simulink model "Sanboks_SIMULINK_v0_4"  (R2021a)
settings: Solver=ode45  StartTime=0  StopTime=1600  FixedStep=1  RelTol=1e-4
InitFcn:
  | Acc_x=0;
undefined symbols (not defined in the file): achievable_velocity, air_density, car_mass, center_of_gravity, coefficient_rolling_resistance, conti_PID, conti_rpm, conti_torque, current, distance, drag_coefficient, final_drivetrain_efficiency, front_braking_torque, front_frequency, front_motion_ratio, front_tire_rate, front_trackwidth, frontal_area, gear_ratio, grade_of_track, gravity, h1f, h1r, hf, hr, long_friction, no_laps, no_of_motors, peak_PID, peak_rpm, peak_torque, Rear_braking_torque, rear_frequency, rear_motion_ratio, rear_tire_rate, rear_trackwidth, rear_weight_distribution, reference_steering_angle, rho, rot_mass, start_time_for_peak, steering_ratio, supply_voltage, tire_radius, track_length, wheelbase, x_leng
libraries: simulink x2, pid_lib x2
settings Model: Creator=Swapnil Mane  LastModifiedBy=rk
settings SolverCC: MaxConsecutiveMinStep=auto  ZeroCrossAlgorithm=Adaptive  AlgebraicLoopSolver=TrustRegion  SolverResetMethod=Robust
settings DebuggingCC: AlgebraicLoopMsg=none  MaskedZcDiagnostic=none  IgnoredZcDiagnostic=none  SFMachineParentedDataDiag=warning

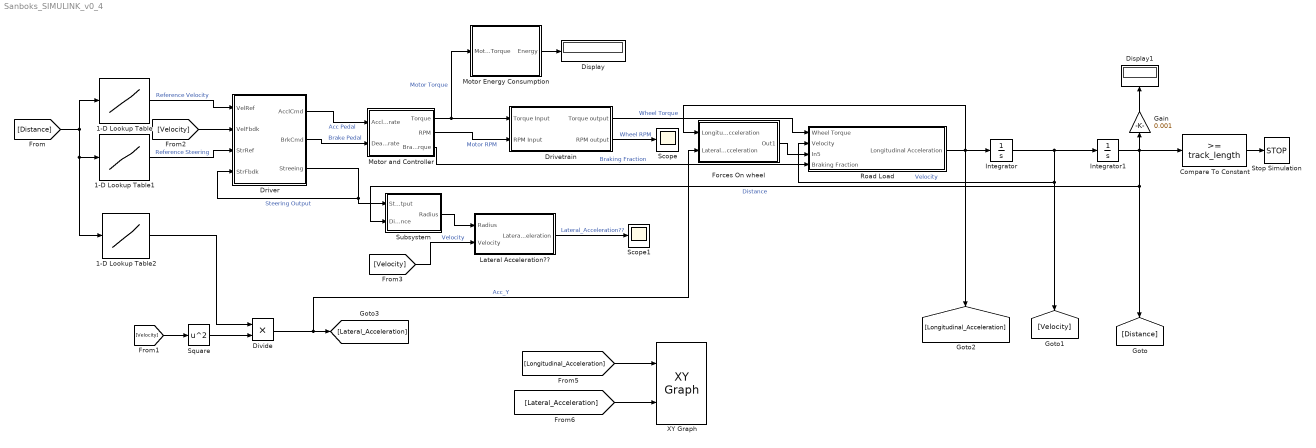
== system Sanboks_SIMULINK_v0_4 ==
  1-D Lookup Table : Lookup_n-D  NumberOfTableDimensions=1  BreakpointsForDimension1=distance(1:2:x_leng*no_laps)  Table=achievable_velocity  InternalRulePriority=Speed  RndMeth=Simplest  InputSameDT=on
  1-D Lookup Table1 : Lookup_n-D  NumberOfTableDimensions=1  BreakpointsForDimension1=distance(1:x_leng*no_laps)  Table=reference_steering_angle  InternalRulePriority=Speed  RndMeth=Simplest  InputSameDT=on
  1-D Lookup Table2 : Lookup_n-D  NumberOfTableDimensions=1  BreakpointsForDimension1=distance(1:2:x_leng*no_laps)  Table=rho  InternalRulePriority=Speed  RndMeth=Simplest  InputSameDT=on
  Compare To Constant : simulink/Logic and Bit Operations/Compare To Constant  relop=>=  const=track_length  OutDataTypeStr=boolean
  Display : Display
  Display1 : Display
  Divide : Product  Inputs=**
  Driver : Subsystem
      mask Display: image('$imagefile'); % Use "Edit Image" on toolstrip to change.
  Drivetrain : Subsystem
      mask Display: image('$imagefile'); % Use "Edit Image" on toolstrip to change.
  Forces On wheel : Subsystem
  Gain : Gain  Gain=0.001
  Integrator : Integrator
  Integrator1 : Integrator
  Lateral Acceleration?? : Subsystem
  Motor Energy Consumption : Subsystem
  Motor and Controller : Subsystem
      mask Display: image('$imagefile'); % Use "Edit Image" on toolstrip to change.
  Road Load : Subsystem
  Scope : Scope
  Scope1 : Scope
  Square : Math  Operator=square  SaturateOnIntegerOverflow=on
  Stop Simulation : Stop
  Subsystem : Subsystem
  XY Graph : simulink/Sinks/XY Graph  xmin=-20  xmax=20  ymin=-20  ymax=20  st=-1
  wires:
  Driver/1(AcclCmd) -> Motor and Controller/1(Acclerate)  "Acc Pedal"
  Motor and Controller/1(Torque) -> Drivetrain/1(Torque Input), Motor Energy Consumption/1(Motor Torque)  "Motor Torque"
  Motor and Controller/2(" RPM") -> Drivetrain/2(RPM Input)  "Motor RPM"
  Driver/2(BrkCmd) -> Motor and Controller/2(Deaccelerate)  "Brake Pedal"
  Compare To Constant/1 -> Stop Simulation/1
  Integrator1/1 -> Compare To Constant/1, Gain/1, [Distance], Subsystem/2(Distance)  "Distance"
  1-D Lookup Table/1 -> Driver/1(VelRef)  "Reference Velocity"
  Integrator/1 -> Integrator1/1, Road Load/2(Velocity), [Velocity]  "Velocity"
  1-D Lookup Table1/1 -> Driver/3(StrRef)  "Reference Steering"
  Driver/3(Streeing) -> Driver/4(StrFbdk), Subsystem/1(Steering Output)  "Steering Output"
  [Velocity] -> Driver/2(VelFbdk)
  [Velocity] -> Lateral Acceleration??/2(Velocity)  "Velocity"
  [Lateral_Acceleration] -> XY Graph/2
  [Longitudinal_Acceleration] -> XY Graph/1
  Subsystem/1(Radius) -> Lateral Acceleration??/1(Radius)
  Motor Energy Consumption/1(Energy) -> Display/1
  Drivetrain/2(RPM output) -> Scope/1  "Wheel RPM"
  [Distance] -> 1-D Lookup Table2/1, 1-D Lookup Table1/1, 1-D Lookup Table/1
  Gain/1 -> Display1/1
  Road Load/1(Longitudinal Acceleration) -> Forces On wheel/1(Longitunal Acceleration), [Longitudinal_Acceleration], Integrator/1
  Drivetrain/1(Torque output) -> Road Load/1(Wheel Torque)  "Wheel Torque"
  Forces On wheel/1(Out1) -> Road Load/3(In5)
  Motor and Controller/3(Braking Torque) -> Road Load/4(Braking Fraction)  "Braking Fraction"
  1-D Lookup Table2/1 -> Divide/1
  [Velocity] -> Square/1
  Square/1 -> Divide/2
  Divide/1 -> Forces On wheel/2(Lateral_Acceleration), [Lateral_Acceleration]  "Acc_Y"
  Lateral Acceleration??/1(Lateral_Acceleration) -> Scope1/1  "Lateral_Acceleration??"

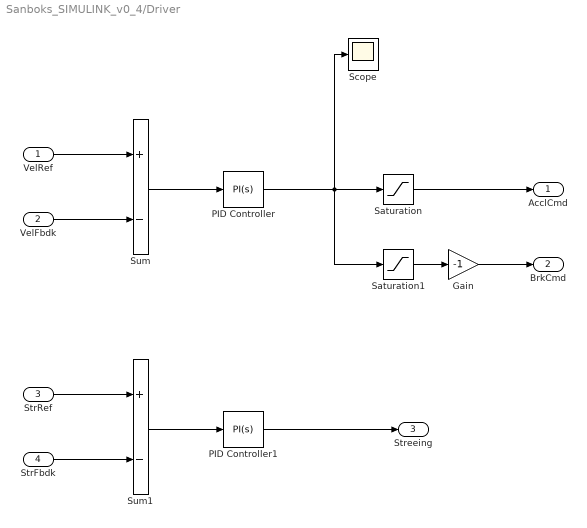
== system Sanboks_SIMULINK_v0_4/Driver ==
  VelRef : Inport
  VelFbdk : Inport  Port=2
  StrRef : Inport  Port=3
  StrFbdk : Inport  Port=4
  Gain : Gain  Gain=-1
  PID Controller : pid_lib/PID Controller  Controller=PI  Form=Parallel  TimeDomain=Continuous-time  UseExternalTs=off  SampleTime=-1  IntegratorMethod=Forward Euler  FilterMethod=Forward Euler  ControllerParametersSource=internal  P=1  I=0  D=0  UseFilter=on  N=10  TunerSelectOption=Transfer Function Based (PID Tuner App)  InitialConditionSource=internal  InitialConditionForIntegrator=0  InitialConditionForFilter=0  DifferentiatorICPrevScaledInput=0  ExternalReset=none  TrackingMode=off  Kt=1  LimitOutput=off  SatLimitsSource=internal  UpperSaturationLimit=inf  LowerSaturationLimit=-inf  LinearizeAsGain=on  AntiWindupMode=none  Kb=1  POutMin=[]  POutMax=[]  IOutMin=[]  IOutMax=[]  DOutMin=[]  DOutMax=[]  NOutMin=[]  NOutMax=[]  SumOutMin=[]  SumOutMax=[]  SaturationOutMin=[]  SaturationOutMax=[]  PParamMin=[]  PParamMax=[]  IParamMin=[]  IParamMax=[]  DParamMin=[]  DParamMax=[]  NParamMin=[]  NParamMax=[]  KbParamMin=[]  KbParamMax=[]  KtParamMin=[]  KtParamMax=[]  KbOutMin=[]  KbOutMax=[]  KtOutMin=[]  KtOutMax=[]  IntegratorOutMin=[]  IntegratorOutMax=[]  FilterOutMin=[]  FilterOutMax=[]  SumI1OutMin=[]  SumI1OutMax=[]  SumI2OutMin=[]  SumI2OutMax=[]  SumI3OutMin=[]  SumI3OutMax=[]  SumI4OutMin=[]  SumI4OutMax=[]  SumDOutMin=[]  SumDOutMax=[]  DifferentiatorOutMin=[]  DifferentiatorOutMax=[]  FilterDiffOutCoefMin=[]  FilterDiffOutCoefMax=[]  ReciprocalOutMin=[]  ReciprocalOutMax=[]  SumDenOutMin=[]  SumDenOutMax=[]  SumNumOutMin=[]  SumNumOutMax=[]  DivideOutMin=[]  DivideOutMax=[]  UdiffTsProdOutMin=[]  UdiffTsProdOutMax=[]  NTsProdOutMin=[]  NTsProdOutMax=[]  UintegralTsProdOutMin=[]  UintegralTsProdOutMax=[]  UngainTsProdOutMin=[]  UngainTsProdOutMax=[]  IntegratorContinuousStateAttributes=''  IntegratorStateMustResolveToSignalObject=off  IntegratorRTWStateStorageClass=Auto  FilterContinuousStateAttributes=''  FilterStateMustResolveToSignalObject=off  FilterRTWStateStorageClass=Auto  ParallelPVariant=InternalParameters  IdealPVariant=Disabled  IVariant=InternalParameters  DVariant=Disabled  IntegratorVariant=Continuous  SatVariant=Disabled  AWVariant=Passthrough  PCopyVariant=Disabled  TRVariant=Disabled  FdbkBlocksVariant=Forward  IdealPFdbkVariant=Disabled  SatFdbkVariant=Disabled  DerivativeFilterVariant=Disabled  NVariant=Disabled  NCopyVariant=Disabled_SignalSpec  FilterICVariant=Disabled  IntegratorICVariant=InternalICs  ExternalResetVariant=Disabled  TRSumVariant=Passthrough  SumFdbkVariant=Disabled  SumVariant=Sum_PI  TsampFilterVariant=InternalTs  TsampNgainVariant=Passthrough  TsampIntegralVariant=Passthrough  ExternalSaturationOutDataTypeStr=Inherit: Same as second input
  PID Controller1 : pid_lib/PID Controller  Controller=PI  Form=Parallel  TimeDomain=Continuous-time  UseExternalTs=off  SampleTime=-1  IntegratorMethod=Forward Euler  FilterMethod=Forward Euler  ControllerParametersSource=internal  P=2  I=1  D=0  UseFilter=on  N=10  TunerSelectOption=Transfer Function Based (PID Tuner App)  InitialConditionSource=internal  InitialConditionForIntegrator=0  InitialConditionForFilter=0  DifferentiatorICPrevScaledInput=0  ExternalReset=none  TrackingMode=off  Kt=1  LimitOutput=off  SatLimitsSource=internal  UpperSaturationLimit=inf  LowerSaturationLimit=-inf  LinearizeAsGain=on  AntiWindupMode=none  Kb=1  POutMin=[]  POutMax=[]  IOutMin=[]  IOutMax=[]  DOutMin=[]  DOutMax=[]  NOutMin=[]  NOutMax=[]  SumOutMin=[]  SumOutMax=[]  SaturationOutMin=[]  SaturationOutMax=[]  PParamMin=[]  PParamMax=[]  IParamMin=[]  IParamMax=[]  DParamMin=[]  DParamMax=[]  NParamMin=[]  NParamMax=[]  KbParamMin=[]  KbParamMax=[]  KtParamMin=[]  KtParamMax=[]  KbOutMin=[]  KbOutMax=[]  KtOutMin=[]  KtOutMax=[]  IntegratorOutMin=[]  IntegratorOutMax=[]  FilterOutMin=[]  FilterOutMax=[]  SumI1OutMin=[]  SumI1OutMax=[]  SumI2OutMin=[]  SumI2OutMax=[]  SumI3OutMin=[]  SumI3OutMax=[]  SumI4OutMin=[]  SumI4OutMax=[]  SumDOutMin=[]  SumDOutMax=[]  DifferentiatorOutMin=[]  DifferentiatorOutMax=[]  FilterDiffOutCoefMin=[]  FilterDiffOutCoefMax=[]  ReciprocalOutMin=[]  ReciprocalOutMax=[]  SumDenOutMin=[]  SumDenOutMax=[]  SumNumOutMin=[]  SumNumOutMax=[]  DivideOutMin=[]  DivideOutMax=[]  UdiffTsProdOutMin=[]  UdiffTsProdOutMax=[]  NTsProdOutMin=[]  NTsProdOutMax=[]  UintegralTsProdOutMin=[]  UintegralTsProdOutMax=[]  UngainTsProdOutMin=[]  UngainTsProdOutMax=[]  IntegratorContinuousStateAttributes=''  IntegratorStateMustResolveToSignalObject=off  IntegratorRTWStateStorageClass=Auto  FilterContinuousStateAttributes=''  FilterStateMustResolveToSignalObject=off  FilterRTWStateStorageClass=Auto  ParallelPVariant=InternalParameters  IdealPVariant=Disabled  IVariant=InternalParameters  DVariant=Disabled  IntegratorVariant=Continuous  SatVariant=Disabled  AWVariant=Passthrough  PCopyVariant=Disabled  TRVariant=Disabled  FdbkBlocksVariant=Forward  IdealPFdbkVariant=Disabled  SatFdbkVariant=Disabled  DerivativeFilterVariant=Disabled  NVariant=Disabled  NCopyVariant=Disabled_SignalSpec  FilterICVariant=Disabled  IntegratorICVariant=InternalICs  ExternalResetVariant=Disabled  TRSumVariant=Passthrough  SumFdbkVariant=Disabled  SumVariant=Sum_PI  TsampFilterVariant=InternalTs  TsampNgainVariant=Passthrough  TsampIntegralVariant=Passthrough  ExternalSaturationOutDataTypeStr=Inherit: Same as second input
  Saturation : Saturate  UpperLimit=1  LowerLimit=0
  Saturation1 : Saturate  UpperLimit=0  LowerLimit=-1
  Scope : Scope
  Sum : Sum  Inputs=+-
  Sum1 : Sum  Inputs=+-
  AcclCmd : Outport
  BrkCmd : Outport  Port=2
  Streeing : Outport  Port=3
  wires:
  PID Controller/1 -> Saturation1/1, Saturation/1, Scope/1
  VelFbdk/1 -> Sum/2
  Sum/1 -> PID Controller/1
  VelRef/1 -> Sum/1
  Saturation/1 -> AcclCmd/1
  Gain/1 -> BrkCmd/1
  Saturation1/1 -> Gain/1
  StrRef/1 -> Sum1/1
  Sum1/1 -> PID Controller1/1
  StrFbdk/1 -> Sum1/2
  PID Controller1/1 -> Streeing/1

== system Sanboks_SIMULINK_v0_4/Drivetrain ==
  Torque Input : Inport
  RPM Input : Inport  Port=2
  Divide : Product  Inputs=**/
  Divide1 : Product  Inputs=***
  Final Drivetrain Efficiency : Constant  Value=final_drivetrain_efficiency
  Gear Ratio : Constant  Value=gear_ratio
  Torque output : Outport
  RPM output : Outport  Port=2
  wires:
  Gear Ratio/1 -> Divide/3, Divide1/1
  Final Drivetrain Efficiency/1 -> Divide1/3, Divide/1
  RPM Input/1 -> Divide/2
  Divide/1 -> RPM output/1
  Torque Input/1 -> Divide1/2
  Divide1/1 -> Torque output/1

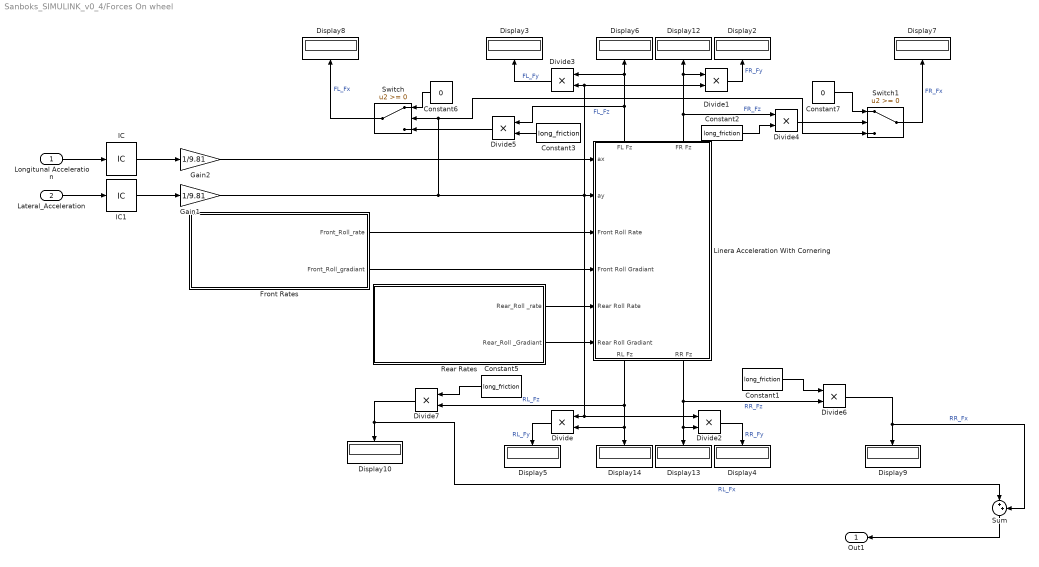
== system Sanboks_SIMULINK_v0_4/Forces On wheel ==
  Longitunal Acceleration : Inport
  Lateral_Acceleration : Inport  Port=2
  Constant{1..3,5} (4 alike) : Constant  Value=long_friction
  Constant6 : Constant  Value=0
  Constant7 : Constant  Value=0
  Display{2..10,12..14} (12 alike) : Display
  Divide{,1..7} (8 alike) : Product  Inputs=**
  Front Rates : Subsystem
  Gain1 : Gain  Gain=1/9.81
  Gain2 : Gain  Gain=1/9.81
  IC : InitialCondition  Value=0
  IC1 : InitialCondition  Value=0
  Linera Acceleration With Cornering : Subsystem
      settings: PortSchema="{\"entries\":[{\"content\":{\"sides\":[{\"content\":{\"connectorIds\":[\"In1\",\"In2\",\"In3\",\"In4\",\"In5\",\"In6\"]},\"type\":\"ConnectorPlacement.EquallySpacedRectSide\",\"uuid\":\"d773b041-193b-40c1-84f4-1820b4697a0f\"},{\"content\":{\"connectorIds\":[],\"side\":\"RIGHT\"},\"type\":\"ConnectorPlacement.EquallySpacedRectSide\",\"uuid\":\"63078260-0e7d-46b5-b894-dfb0cdd11ba9\"},{\"content\":{\"connectorIds\":[\"Out3\",\"Out4\"],\"side\":\"TOP\"},\"type\":\"ConnectorPlacement.EquallySpacedRectSide\",\"uuid\":\"e8ba9282-0130-45e1-8a34-44ae52181d51\"},{\"content\":{\"connectorIds\":[\"Out1\",\"Out2\"],\"side\":\"BOTTOM\"},\"type\":\"ConnectorPlacement.EquallySpacedRectSide\",\"uuid\":\"5bbf88fe-c1d3-4396-8228-1f5368518a99\"},{\"content\":{\"connectorIds\":[],\"side\":\"HIDDEN\"},\"type\":\"ConnectorPlacement.EquallySpacedRectSide\",\"uuid\":\"f592c54a-f6c6-4a08-a46d-6911c26235f2\"}]},\"type\":\"ConnectorPlacement.EquallySpacedConnector\",\"uuid\":\"5d9b9e8e-da8b-47d2-a239-b5c86b3b0142\"}],\"packageUris\":[\"http://schema.mathworks.com/mf0/Connector/R2020b\"],\"version\":\"1.0\"}"
  Rear Rates : Subsystem
  Sum : Sum  Inputs=|++
  Switch : Switch
  Switch1 : Switch
  Out1 : Outport
  wires:
  Switch1/1 -> Display7/1  "FR_Fx"
  Constant2/1 -> Divide4/2
  Constant3/1 -> Divide5/2
  Linera Acceleration With Cornering/2(RR Fz) -> Divide6/2, Divide2/2, Display13/1  "RR_Fz"
  Front Rates/1(Front_Roll_rate) -> Linera Acceleration With Cornering/3(Front Roll Rate)
  Divide6/1 -> Sum/2, Display9/1  "RR_Fx"
  Front Rates/2(Front_Roll_gradiant) -> Linera Acceleration With Cornering/4(Front Roll Gradiant)
  Gain1/1 -> Switch1/2, Switch/2, Linera Acceleration With Cornering/2(ay), Divide3/2, Divide1/2, Divide2/1, Divide/1
  Rear Rates/2(Rear_Roll _Gradiant) -> Linera Acceleration With Cornering/6(Rear Roll Gradiant)
  Divide1/1 -> Display2/1  "FR_Fy"
  Linera Acceleration With Cornering/1(RL Fz) -> Divide7/2, Divide/2, Display14/1  "RL_Fz"
  Divide5/1 -> Switch/3
  Constant5/1 -> Divide7/1
  Rear Rates/1(Rear_Roll _rate) -> Linera Acceleration With Cornering/5(Rear Roll Rate)
  Linera Acceleration With Cornering/3(" FL Fz") -> Divide5/1, Display6/1, Divide3/1  "FL_Fz"
  Divide4/1 -> Switch1/3
  Divide7/1 -> Display10/1, Sum/1  "RL_Fx"
  Linera Acceleration With Cornering/4(FR Fz) -> Divide1/1, Display12/1, Divide4/1  "FR_Fz"
  Gain2/1 -> Linera Acceleration With Cornering/1(ax)
  Divide3/1 -> Display3/1  "FL_Fy"
  Constant1/1 -> Divide6/1
  Divide/1 -> Display5/1  "RL_Fy"
  Constant6/1 -> Switch/1
  Divide2/1 -> Display4/1  "RR_Fy"
  Sum/1 -> Out1/1
  Switch/1 -> Display8/1  "FL_Fx"
  Constant7/1 -> Switch1/1
  IC/1 -> Gain2/1
  IC1/1 -> Gain1/1
  Longitunal Acceleration/1 -> IC/1
  Lateral_Acceleration/1 -> IC1/1

== system Sanboks_SIMULINK_v0_4/Lateral Acceleration?? ==
  Radius : Inport
  Velocity : Inport  Port=2
  Divide2 : Product  Inputs=**/
  Scope13 : Scope
  Lateral_Acceleration : Outport
  wires:
  Divide2/1 -> Lateral_Acceleration/1, Scope13/1
  Radius/1 -> Divide2/3
  Velocity/1 -> Divide2/2, Divide2/1

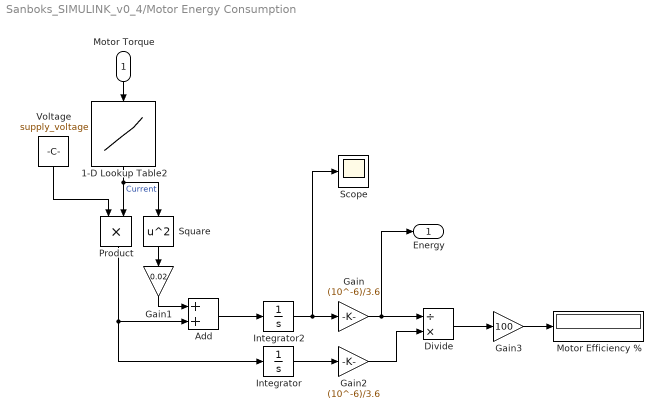
== system Sanboks_SIMULINK_v0_4/Motor Energy Consumption ==
  Motor Torque : Inport
  1-D Lookup Table2 : Lookup_n-D  NumberOfTableDimensions=1  BreakpointsForDimension1=peak_torque  Table=current  InternalRulePriority=Speed  RndMeth=Simplest  InputSameDT=on
  Add : Sum
  Divide : Product  Inputs=/*
  Gain : Gain  Gain=(10^-6)/3.6
  Gain1 : Gain  Gain=0.02
  Gain2 : Gain  Gain=(10^-6)/3.6
  Gain3 : Gain  Gain=100
  Integrator : Integrator
  Integrator2 : Integrator
  Motor Efficiency % : Display
  Product : Product
  Scope : Scope
  Square : Math  Operator=square  SaturateOnIntegerOverflow=on
  Voltage : Constant  Value=supply_voltage
  Energy : Outport
  wires:
  Product/1 -> Integrator/1, Add/2
  Gain1/1 -> Add/1
  Voltage/1 -> Product/1
  Add/1 -> Integrator2/1
  1-D Lookup Table2/1 -> Product/2, Square/1  "Current"
  Integrator2/1 -> Scope/1, Gain/1
  Motor Torque/1 -> 1-D Lookup Table2/1
  Gain/1 -> Energy/1, Divide/1
  Square/1 -> Gain1/1
  Integrator/1 -> Gain2/1
  Gain2/1 -> Divide/2
  Divide/1 -> Gain3/1
  Gain3/1 -> Motor Efficiency %/1

== system Sanboks_SIMULINK_v0_4/Motor and Controller ==
  Acclerate : Inport
  Deaccelerate : Inport  Port=2
  Motor : Subsystem
  Motor Controller : Subsystem
  Scope : Scope
  Torque : Outport
  " RPM" : Outport  Port=2
  Braking Torque : Outport  Port=3
  wires:
  Acclerate/1 -> Motor Controller/1(Acclerate)
  Deaccelerate/1 -> Motor Controller/2(Deaccelerate)
  Motor Controller/1(Peak) -> Scope/1, Motor/1(Peak)
  Motor Controller/2(Cont) -> Motor/2(Cont)
  Motor/1(Out1) -> " RPM"/1
  Motor/2(Out2) -> Torque/1
  Motor Controller/3(braking torque) -> Braking Torque/1

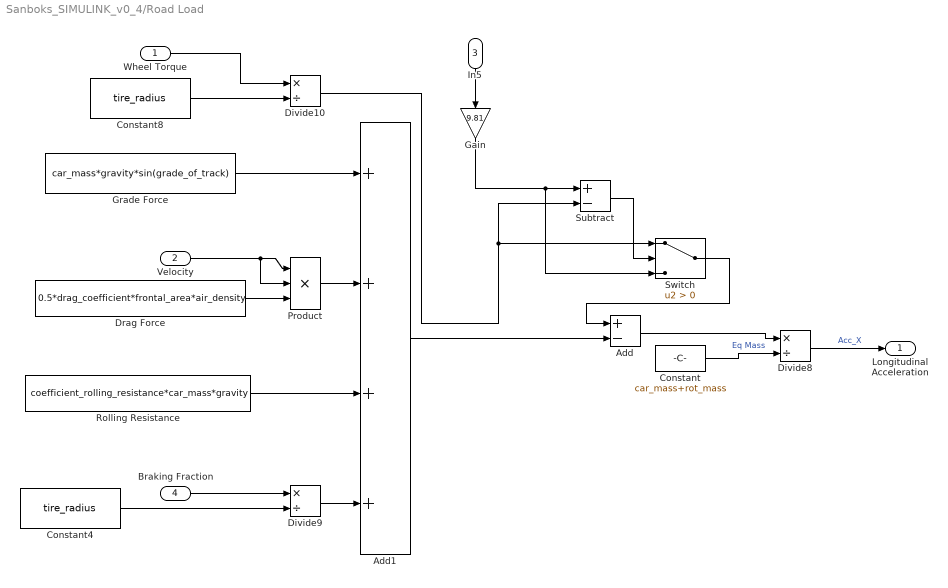
== system Sanboks_SIMULINK_v0_4/Road Load ==
  Wheel Torque : Inport
  Velocity : Inport  Port=2
  In5 : Inport  Port=3
  Braking Fraction : Inport  Port=4
  Add : Sum  Inputs=+-
  Add1 : Sum  Inputs=++++
  Constant : Constant  Value=car_mass+rot_mass
  Constant4 : Constant  Value=tire_radius
  Constant8 : Constant  Value=tire_radius
  Divide10 : Product  Inputs=*/
  Divide8 : Product  Inputs=*/
  Divide9 : Product  Inputs=*/
  Drag Force : Constant  Value=0.5*drag_coefficient*frontal_area*air_density
  Gain : Gain  Gain=9.81
  Grade Force : Constant  Value=car_mass*gravity*sin(grade_of_track)
  Product : Product  Inputs=3
  Rolling Resistance : Constant  Value=coefficient_rolling_resistance*car_mass*gravity
  Subtract : Sum  Inputs=+-
  Switch : Switch  Criteria=u2 > Threshold
  Longitudinal Acceleration : Outport
  wires:
  Drag Force/1 -> Product/3
  Rolling Resistance/1 -> Add1/3
  Product/1 -> Add1/2
  Velocity/1 -> Product/2, Product/1
  Grade Force/1 -> Add1/1
  Divide10/1 -> Switch/1, Subtract/2
  Constant8/1 -> Divide10/2
  Divide9/1 -> Add1/4
  Constant4/1 -> Divide9/2
  Braking Fraction/1 -> Divide9/1
  Wheel Torque/1 -> Divide10/1
  In5/1 -> Gain/1
  Constant/1 -> Divide8/2  "Eq Mass"
  Add1/1 -> Add/2
  Add/1 -> Divide8/1
  Gain/1 -> Switch/3, Subtract/1
  Subtract/1 -> Switch/2
  Switch/1 -> Add/1
  Divide8/1 -> Longitudinal Acceleration/1  "Acc_X"

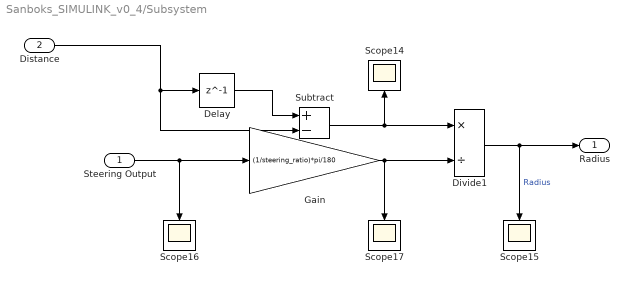
== system Sanboks_SIMULINK_v0_4/Subsystem ==
  Steering Output : Inport
  Distance : Inport  Port=2
  Delay : Delay  DelayLength=1
  Divide1 : Product  Inputs=*/
  Gain : Gain  Gain=(1/steering_ratio)*pi/180
  Scope{14..17} (4 alike) : Scope
  Subtract : Sum  Inputs=+-
  Radius : Outport
  wires:
  Distance/1 -> Subtract/2, Delay/1
  Gain/1 -> Divide1/2, Scope17/1
  Subtract/1 -> Divide1/1, Scope14/1
  Divide1/1 -> Scope15/1, Radius/1  "Radius"
  Steering Output/1 -> Gain/1, Scope16/1
  Delay/1 -> Subtract/1

== system Sanboks_SIMULINK_v0_4/Forces On wheel/Front Rates ==
  Constant1 : Constant  Value=front_trackwidth^2*(pi()/360)
  Divide2 : Product  Inputs=**
  Divide5 : Product  Inputs=*/
  Front Left1 : Constant  Value=((1-rear_weight_distribution)*car_mass/2)*2*9.81*h1f
  Front Roll Rate : Display
  Front Roll rate : Display
  Front_ride_rate : Subsystem
  Front_Roll_rate : Outport
  Front_Roll_gradiant : Outport  Port=2
  wires:
  Divide2/1 -> Front Roll rate/1, Divide5/2, Front_Roll_rate/1  "Front_Roll _rate"
  Divide5/1 -> Front_Roll_gradiant/1, Front Roll Rate/1  "Roll Gradiant"
  Front_ride_rate/1(front wheel rate) -> Divide2/2
  Constant1/1 -> Divide2/1
  Front Left1/1 -> Divide5/1

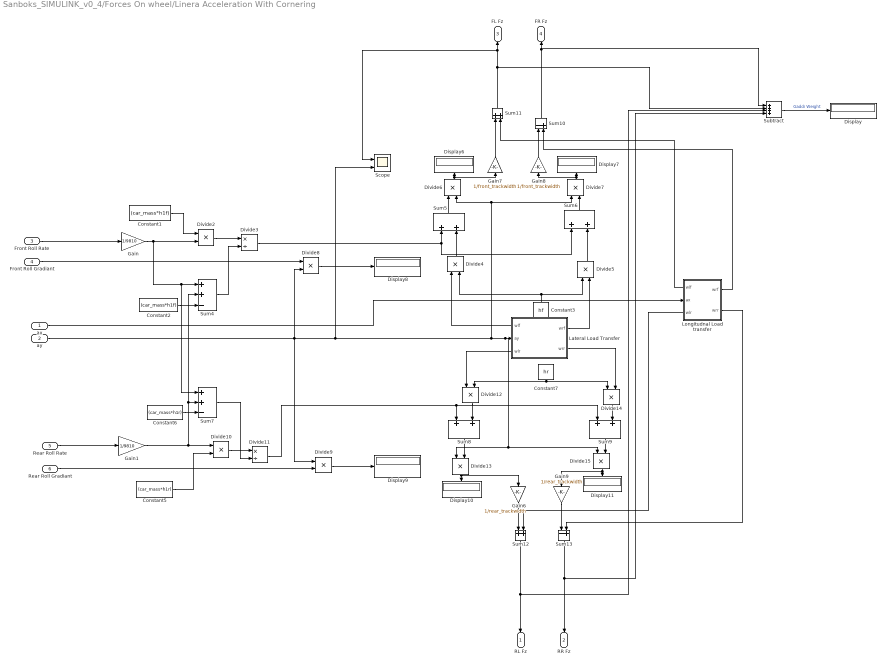
== system Sanboks_SIMULINK_v0_4/Forces On wheel/Linera Acceleration With Cornering ==
  ax : Inport
  ay : Inport  Port=2
  Front Roll Rate : Inport  Port=3
  Front Roll Gradiant : Inport  Port=4
  Rear Roll Rate : Inport  Port=5
  Rear Roll Gradiant : Inport  Port=6
  Constant1 : Constant  Value=(car_mass*h1f)
  Constant2 : Constant  Value=(car_mass*h1f)
  Constant3 : Constant  Value=hf
  Constant5 : Constant  Value=(car_mass*h1r)
  Constant6 : Constant  Value=(car_mass*h1r)
  Constant7 : Constant  Value=hr
  Display{,6..11} (7 alike) : Display
  Divide{2,4..10,12..15} (12 alike) : Product  Inputs=**
  Divide11 : Product  Inputs=*/
  Divide3 : Product  Inputs=*/
  Gain : Gain  Gain=1/9810
  Gain1 : Gain  Gain=1/9810
  Gain6 : Gain  Gain=1/rear_trackwidth
  Gain7 : Gain  Gain=1/front_trackwidth
  Gain8 : Gain  Gain=1/front_trackwidth
  Gain9 : Gain  Gain=1/rear_trackwidth
  Lateral Load Transfer : Subsystem
      settings: PortSchema="{\"entries\":[{\"content\":{\"sides\":[{\"content\":{\"connectorIds\":[\"Out3\",\"In1\",\"Out4\"]},\"type\":\"ConnectorPlacement.EquallySpacedRectSide\",\"uuid\":\"3c1d5b41-10a3-449f-a4be-56571e187b1f\"},{\"content\":{\"connectorIds\":[\"Out1\",\"Out2\"],\"side\":\"RIGHT\"},\"type\":\"ConnectorPlacement.EquallySpacedRectSide\",\"uuid\":\"93fd1353-89e6-4160-b3cc-079c084db1dd\"},{\"content\":{\"connectorIds\":[],\"side\":\"TOP\"},\"type\":\"ConnectorPlacement.EquallySpacedRectSide\",\"uuid\":\"03e3719f-7b8c-4e64-81ea-821c7eb402ea\"},{\"content\":{\"connectorIds\":[],\"side\":\"HIDDEN\"},\"type\":\"ConnectorPlacement.EquallySpacedRectSide\",\"uuid\":\"b030b923-f911-4f6e-b446-7b237ff20193\"}]},\"type\":\"ConnectorPlacement.EquallySpacedConnector\",\"uuid\":\"a6aa80b4-4da8-4715-a122-7a3096c60bae\"}],\"packageUris\":[\"http://schema.mathworks.com/mf0/Connector/R2020b\"],\"version\":\"1.0\"}"
  Longitudnal Load transfer : Subsystem
      settings: PortSchema="{\"entries\":[{\"content\":{\"sides\":[{\"content\":{\"connectorIds\":[\"Out3\",\"In1\",\"Out4\"]},\"type\":\"ConnectorPlacement.EquallySpacedRectSide\",\"uuid\":\"0af3428f-ed27-4406-8056-80f0213c93e8\"},{\"content\":{\"connectorIds\":[\"Out1\",\"Out2\"],\"side\":\"RIGHT\"},\"type\":\"ConnectorPlacement.EquallySpacedRectSide\",\"uuid\":\"4433f412-cc8d-4119-9301-f989dff2ced8\"},{\"content\":{\"connectorIds\":[],\"side\":\"TOP\"},\"type\":\"ConnectorPlacement.EquallySpacedRectSide\",\"uuid\":\"6e72867b-bd7e-4656-b901-a84940f85d37\"},{\"content\":{\"connectorIds\":[],\"side\":\"HIDDEN\"},\"type\":\"ConnectorPlacement.EquallySpacedRectSide\",\"uuid\":\"6dc56d18-9c05-4bcc-a4c3-9a4105b122ee\"}]},\"type\":\"ConnectorPlacement.EquallySpacedConnector\",\"uuid\":\"ad876c47-21c6-419e-a299-8440669eb380\"}],\"packageUris\":[\"http://schema.mathworks.com/mf0/Connector/R2020b\"],\"version\":\"1.0\"}"
  Scope : Scope  NumInputPorts=2
  Subtract : Sum  Inputs=++++
  Sum10 : Sum  Inputs=-+
  Sum{5..6,8..9,11..12} (6 alike) : Sum
  Sum13 : Sum  Inputs=-+
  Sum4 : Sum  Inputs=++-
  Sum7 : Sum  Inputs=++-
  RL Fz : Outport
  RR Fz : Outport  Port=2
  " FL Fz" : Outport  Port=3
  FR Fz : Outport  Port=4
  wires:
  Lateral Load Transfer/3(wlf) -> Divide4/1
  Lateral Load Transfer/4(wlr) -> Divide12/1
  Lateral Load Transfer/1(wrf) -> Divide5/1
  Divide5/1 -> Sum6/2
  Divide7/1 -> Gain8/1, Display7/1
  Divide6/1 -> Gain7/1, Display6/1
  Divide13/1 -> Gain6/1, Display10/1
  Lateral Load Transfer/2(wrr) -> Divide14/2
  Gain9/1 -> Sum13/1
  Divide15/1 -> Gain9/1, Display11/1
  Constant7/1 -> Divide14/1, Divide12/2
  Gain7/1 -> Sum11/1
  Sum8/1 -> Divide13/2
  Sum5/1 -> Divide6/1
  Longitudnal Load transfer/2(wrr) -> Sum13/2
  Constant3/1 -> Divide5/2, Divide4/2
  Divide12/1 -> Sum8/2
  Divide11/1 -> Sum9/1, Sum8/1
  Divide3/1 -> Sum5/1, Sum6/1
  Sum6/1 -> Divide7/2
  Divide4/1 -> Sum5/2
  Gain8/1 -> Sum10/1
  Divide14/1 -> Sum9/2
  Sum9/1 -> Divide15/2
  Longitudnal Load transfer/4(wlr) -> Sum12/2
  Longitudnal Load transfer/3(wlf) -> Sum11/2
  Longitudnal Load transfer/1(wrf) -> Sum10/2
  Gain6/1 -> Sum12/1
  ax/1 -> Longitudnal Load transfer/1(ax)
  Sum4/1 -> Divide3/2
  Sum7/1 -> Divide11/2
  Constant6/1 -> Sum7/3
  Gain1/1 -> Divide10/1, Sum7/2, Sum4/2
  Constant1/1 -> Divide2/1
  Constant5/1 -> Divide10/2
  Divide9/1 -> Display9/1
  Constant2/1 -> Sum4/3
  Divide2/1 -> Divide3/1
  Divide10/1 -> Divide11/1
  Divide8/1 -> Display8/1
  Gain/1 -> Sum7/1, Sum4/1, Divide2/2
  Front Roll Gradiant/1 -> Divide8/1
  ay/1 -> Scope/2, Divide13/1, Divide15/1, Lateral Load Transfer/1(ay), Divide6/2, Divide7/1, Divide9/1, Divide8/2
  Rear Roll Gradiant/1 -> Divide9/2
  Front Roll Rate/1 -> Gain/1
  Rear Roll Rate/1 -> Gain1/1
  Sum10/1 -> FR Fz/1, Subtract/1
  Sum12/1 -> Subtract/3, RL Fz/1
  Sum13/1 -> Subtract/4, RR Fz/1
  Sum11/1 -> Subtract/2, Scope/1, " FL Fz"/1
  Subtract/1 -> Display/1  "Gaddi Weight"

== system Sanboks_SIMULINK_v0_4/Forces On wheel/Rear Rates ==
  Constant2 : Constant  Value=rear_trackwidth^2*(pi()/360)
  Divide3 : Product  Inputs=**
  Divide4 : Product  Inputs=*/
  Rates : Constant  Value=((rear_weight_distribution)*car_mass/2)*2*9.81*h1r
  Rear Roll Rate : Display
  Rear_Roll_Gradiant : Display
  Rear_ride_rate : Subsystem
  Rear_Roll _rate : Outport
  Rear_Roll _Gradiant : Outport  Port=2
  wires:
  Divide4/1 -> Rear_Roll _Gradiant/1, Rear_Roll_Gradiant/1  "Rear Roll Gradiant"
  Rates/1 -> Divide4/1
  Rear_ride_rate/1(Rear wheel rate) -> Divide3/2
  Constant2/1 -> Divide3/1
  Divide3/1 -> Rear_Roll _rate/1, Divide4/2, Rear Roll Rate/1  "Rea_Roll _rate"

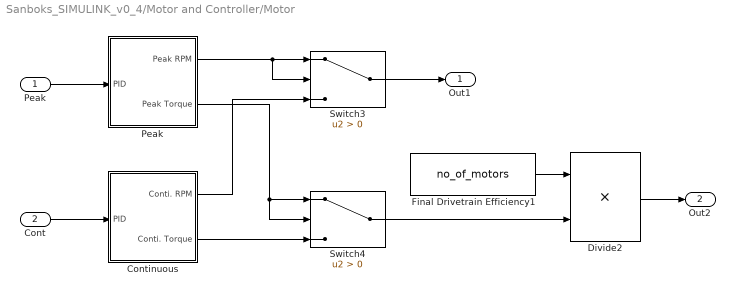
== system Sanboks_SIMULINK_v0_4/Motor and Controller/Motor ==
  Peak : Inport
  Cont : Inport  Port=2
  Continuous : Subsystem
  Divide2 : Product  Inputs=**
  Final Drivetrain Efficiency1 : Constant  Value=no_of_motors
  "Peak " : Subsystem
  Switch3 : Switch  Criteria=u2 > Threshold
  Switch4 : Switch  Criteria=u2 > Threshold
  Out1 : Outport
  Out2 : Outport  Port=2
  wires:
  Cont/1 -> Continuous/1(PID)
  "Peak "/2(Peak Torque) -> Switch4/2, Switch4/1
  "Peak "/1(Peak RPM) -> Switch3/2, Switch3/1
  Continuous/1(Conti. RPM) -> Switch3/3
  Switch3/1 -> Out1/1
  Peak/1 -> "Peak "/1(PID)
  Continuous/2(Conti. Torque) -> Switch4/3
  Switch4/1 -> Divide2/2
  Final Drivetrain Efficiency1/1 -> Divide2/1
  Divide2/1 -> Out2/1

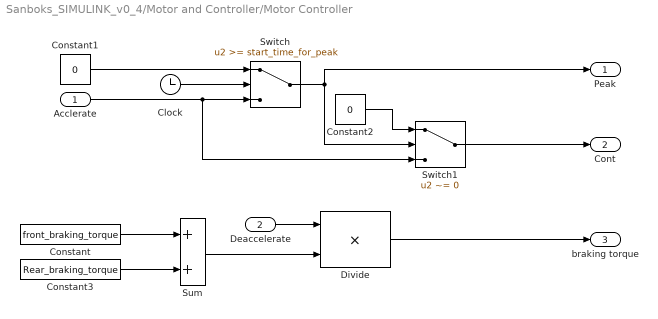
== system Sanboks_SIMULINK_v0_4/Motor and Controller/Motor Controller ==
  Acclerate : Inport
  Deaccelerate : Inport  Port=2
  Clock : Clock
  Constant : Constant  Value=front_braking_torque
  Constant1 : Constant  Value=0
  Constant2 : Constant  Value=0
  Constant3 : Constant  Value=Rear_braking_torque
  Divide : Product  Inputs=**
  Sum : Sum
  Switch : Switch  Threshold=start_time_for_peak
  Switch1 : Switch  Criteria=u2 ~= 0
  Peak : Outport
  Cont : Outport  Port=2
  braking torque : Outport  Port=3
  wires:
  Acclerate/1 -> Switch/3, Switch1/3
  Switch/1 -> Peak/1, Switch1/2
  Switch1/1 -> Cont/1
  Deaccelerate/1 -> Divide/1
  Divide/1 -> braking torque/1
  Constant3/1 -> Sum/2
  Constant/1 -> Sum/1
  Sum/1 -> Divide/2
  Clock/1 -> Switch/2
  Constant1/1 -> Switch/1
  Constant2/1 -> Switch1/1

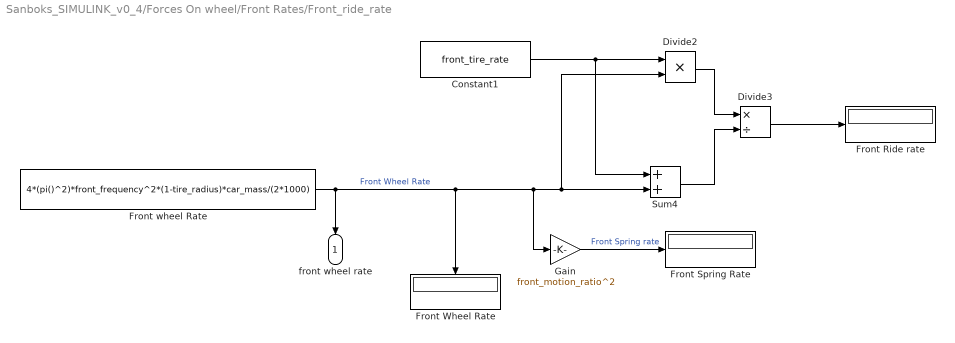
== system Sanboks_SIMULINK_v0_4/Forces On wheel/Front Rates/Front_ride_rate ==
  Constant1 : Constant  Value=front_tire_rate
  Divide2 : Product  Inputs=**
  Divide3 : Product  Inputs=*/
  Front Ride rate : Display
  Front Spring Rate : Display
  Front Wheel Rate : Display
  Front wheel Rate : Constant  Value=4*(pi()^2)*front_frequency^2*(1-tire_radius)*car_mass/(2*1000)
  Gain : Gain  Gain=front_motion_ratio^2
  Sum4 : Sum
  front wheel rate : Outport
  wires:
  Front wheel Rate/1 -> Gain/1, Divide2/2, Sum4/2, Front Wheel Rate/1, front wheel rate/1  "Front Wheel Rate"
  Gain/1 -> Front Spring Rate/1  "Front Spring rate"
  Divide2/1 -> Divide3/1
  Constant1/1 -> Divide2/1, Sum4/1
  Sum4/1 -> Divide3/2
  Divide3/1 -> Front Ride rate/1

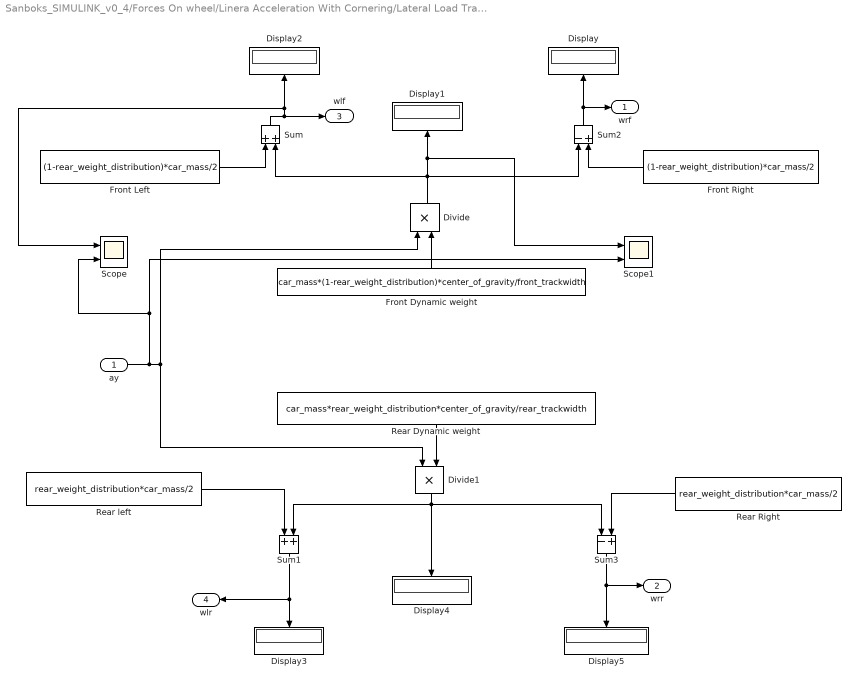
== system Sanboks_SIMULINK_v0_4/Forces On wheel/Linera Acceleration With Cornering/Lateral Load Transfer ==
  ay : Inport
  Display{,1..5} (6 alike) : Display
  Divide : Product  Inputs=**
  Divide1 : Product  Inputs=**
  Front Dynamic weight : Constant  Value=car_mass*(1-rear_weight_distribution)*center_of_gravity/front_trackwidth
  Front Left : Constant  Value=(1-rear_weight_distribution)*car_mass/2
  Front Right : Constant  Value=(1-rear_weight_distribution)*car_mass/2
  Rear Dynamic weight : Constant  Value=car_mass*rear_weight_distribution*center_of_gravity/rear_trackwidth
  Rear Right : Constant  Value=rear_weight_distribution*car_mass/2
  Rear left : Constant  Value=rear_weight_distribution*car_mass/2
  Scope : Scope  NumInputPorts=2
  Scope1 : Scope  NumInputPorts=2
  Sum : Sum
  Sum1 : Sum
  Sum2 : Sum  Inputs=-+
  Sum3 : Sum  Inputs=-+
  wrf : Outport
  wrr : Outport  Port=2
  wlf : Outport  Port=3
  wlr : Outport  Port=4
  wires:
  Front Left/1 -> Sum/1
  Rear left/1 -> Sum1/1
  ay/1 -> Scope/2, Scope1/2, Divide/1, Divide1/1
  Front Right/1 -> Sum2/2
  Divide1/1 -> Display4/1, Sum3/1, Sum1/2
  Rear Dynamic weight/1 -> Divide1/2
  Rear Right/1 -> Sum3/2
  Divide/1 -> Scope1/1, Display1/1, Sum/2, Sum2/1
  Front Dynamic weight/1 -> Divide/2
  Sum/1 -> Display2/1, Scope/1, wlf/1
  Sum2/1 -> Display/1, wrf/1
  Sum3/1 -> Display5/1, wrr/1
  Sum1/1 -> Display3/1, wlr/1

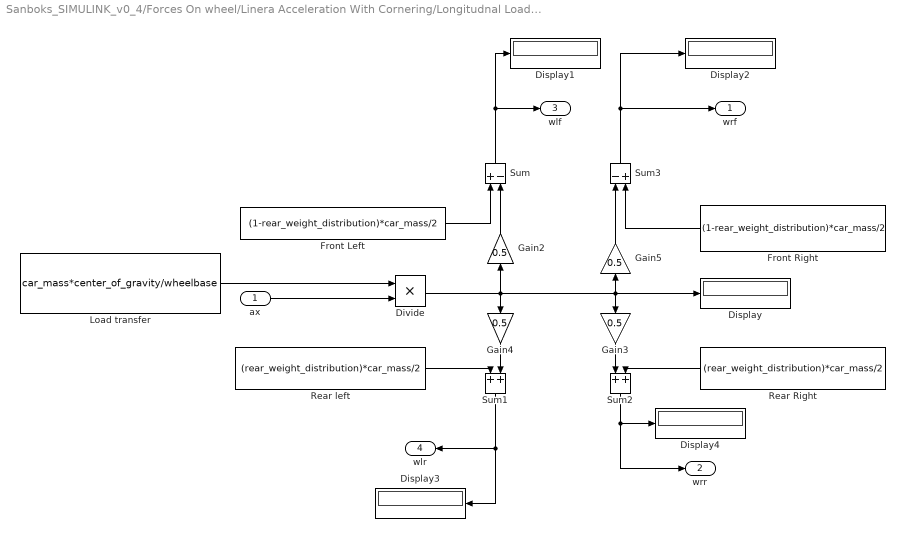
== system Sanboks_SIMULINK_v0_4/Forces On wheel/Linera Acceleration With Cornering/Longitudnal Load transfer ==
  ax : Inport
  Display{,1..4} (5 alike) : Display
  Divide : Product  Inputs=**
  Front Left : Constant  Value=(1-rear_weight_distribution)*car_mass/2
  Front Right : Constant  Value=(1-rear_weight_distribution)*car_mass/2
  Gain{2..5} (4 alike) : Gain  Gain=0.5
  Load transfer : Constant  Value=car_mass*center_of_gravity/wheelbase
  Rear Right : Constant  Value=(rear_weight_distribution)*car_mass/2
  Rear left : Constant  Value=(rear_weight_distribution)*car_mass/2
  Sum : Sum  Inputs=+-
  Sum1 : Sum
  Sum2 : Sum
  Sum3 : Sum  Inputs=-+
  wrf : Outport
  wrr : Outport  Port=2
  wlf : Outport  Port=3
  wlr : Outport  Port=4
  wires:
  Front Left/1 -> Sum/1
  Gain2/1 -> Sum/2
  Gain5/1 -> Sum3/1
  Rear left/1 -> Sum1/1
  Rear Right/1 -> Sum2/2
  Gain3/1 -> Sum2/1
  Gain4/1 -> Sum1/2
  Divide/1 -> Gain4/1, Gain2/1, Gain3/1, Gain5/1, Display/1
  Load transfer/1 -> Divide/1
  Sum/1 -> Display1/1, wlf/1
  Front Right/1 -> Sum3/2
  ax/1 -> Divide/2
  Sum1/1 -> Display3/1, wlr/1
  Sum2/1 -> wrr/1, Display4/1
  Sum3/1 -> wrf/1, Display2/1

== system Sanboks_SIMULINK_v0_4/Forces On wheel/Rear Rates/Rear_ride_rate ==
  Constant2 : Constant  Value=rear_tire_rate
  Divide4 : Product  Inputs=**
  Divide5 : Product  Inputs=*/
  Gain1 : Gain  Gain=rear_motion_ratio^2
  Rear Ride Rate : Display
  Rear Spring Rate : Display
  Rear Wheel Rate : Constant  Value=4*pi()^2*rear_frequency^2*rear_weight_distribution*car_mass/(2*1000)
  Rear_wheel_rate : Display
  Sum5 : Sum
  Rear wheel rate : Outport
  wires:
  Divide5/1 -> Rear Ride Rate/1
  Gain1/1 -> Rear Spring Rate/1  "Rear springrate"
  Constant2/1 -> Sum5/2, Divide4/2
  Sum5/1 -> Divide5/2
  Rear Wheel Rate/1 -> Rear_wheel_rate/1, Rear wheel rate/1, Sum5/1, Divide4/1, Gain1/1
  Divide4/1 -> Divide5/1

== system Sanboks_SIMULINK_v0_4/Motor and Controller/Motor/Continuous ==
  PID : Inport
  1-D Lookup Table : Lookup_n-D  NumberOfTableDimensions=1  BreakpointsForDimension1=conti_PID  Table=conti_rpm  InternalRulePriority=Speed  RndMeth=Simplest  InputSameDT=on
  1-D Lookup Table1 : Lookup_n-D  NumberOfTableDimensions=1  BreakpointsForDimension1=conti_PID  Table=conti_torque  InternalRulePriority=Speed  RndMeth=Simplest  InputSameDT=on
  Conti. RPM : Outport
  Conti. Torque : Outport  Port=2
  wires:
  1-D Lookup Table/1 -> Conti. RPM/1
  PID/1 -> 1-D Lookup Table1/1, 1-D Lookup Table/1
  1-D Lookup Table1/1 -> Conti. Torque/1

== system Sanboks_SIMULINK_v0_4/Motor and Controller/Motor/Peak  ==
  PID : Inport
  1-D Lookup Table2 : Lookup_n-D  NumberOfTableDimensions=1  BreakpointsForDimension1=peak_PID  Table=peak_rpm  InternalRulePriority=Speed  RndMeth=Simplest  InputSameDT=on
  1-D Lookup Table3 : Lookup_n-D  NumberOfTableDimensions=1  BreakpointsForDimension1=peak_PID  Table=peak_torque  InternalRulePriority=Speed  RndMeth=Simplest  InputSameDT=on
  Peak RPM : Outport
  Peak Torque : Outport  Port=2
  wires:
  PID/1 -> 1-D Lookup Table3/1, 1-D Lookup Table2/1
  1-D Lookup Table2/1 -> Peak RPM/1
  1-D Lookup Table3/1 -> Peak Torque/1
